simulink model "lab2_B_gr2159"  (R2022b)
settings: Solver=ode45  StartTime=0.0  StopTime=1  MaxStep=0.001  RelTol=1e-3
settings Model: Creator=gaura  LastModifiedBy=gaura

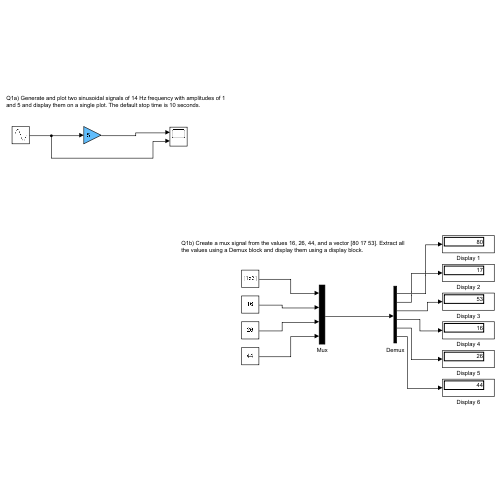
[thumbnail: Simulink's stored preview of the top-level diagram]
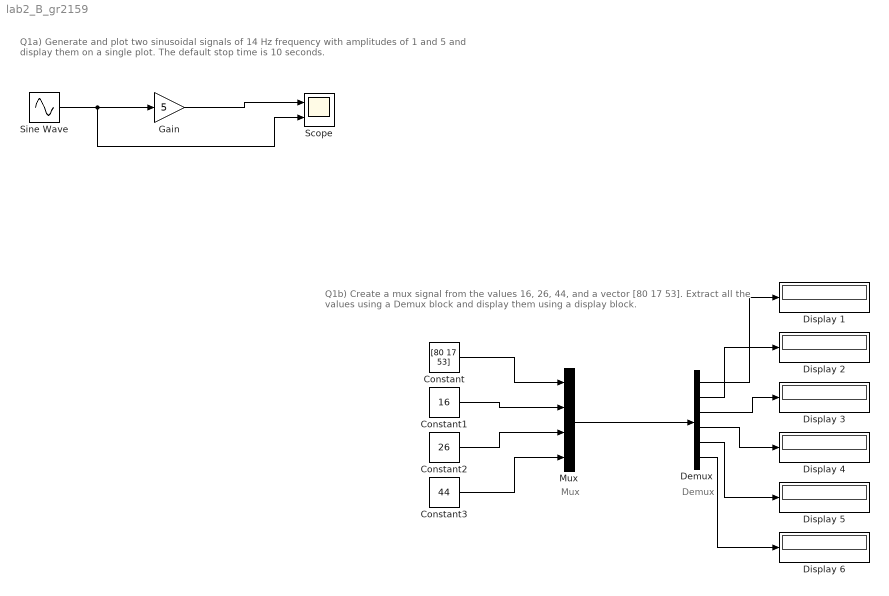
== system lab2_B_gr2159 ==
  note: Demux
  note: Mux
  note: Q1a) Generate and plot two sinusoidal signals of 14 Hz frequency with amplitudes of 1 and 5 and display them on a single plot. The default stop time is 10 seconds.
  note: Q1b) Create a mux signal from the values 16, 26, 44, and a vector [80 17 53]. Extract all the values using a Demux block and display them using a display block.
  Constant : Constant  Value=[80 17 53]
  Constant1 : Constant  Value=16
  Constant2 : Constant  Value=26
  Constant3 : Constant  Value=44
  Demux : Demux  Outputs=6
  Display {1..6} (6 alike) : Display
  Gain : Gain  Gain=5
  Mux : Mux
  Scope : Scope  NumInputPorts=2
  Sine Wave : Sin  Frequency=14*2*pi  SampleTime=0
  wires:
  Sine Wave/1 -> Scope/2, Gain/1
  Gain/1 -> Scope/1
  Constant/1 -> Mux/1
  Constant1/1 -> Mux/2
  Constant2/1 -> Mux/3
  Constant3/1 -> Mux/4
  Mux/1 -> Demux/1
  Demux/1 -> Display 1/1
  Demux/2 -> Display 2/1
  Demux/3 -> Display 3/1
  Demux/4 -> Display 4/1
  Demux/5 -> Display 5/1
  Demux/6 -> Display 6/1
